simulink model "REFvsFI"  (R2023a)
settings: Solver=FixedStepAuto  StartTime=0.0  StopTime=T  RelTol=1e-3  EnableMultiTasking=on
values from neighbouring files (symbols this model uses):
  Ts = 1    [TestDataGen.m]
libraries: My_FI_Operations x114, simulink x2
(part 1 of 5)
settings Model: FPTShortcutValueString='{{},{''BaselineRun'',1,1,1,''BaselineRun'','''',{},''M'',''D'',''''}}'  Creator=kavru  LastModifiedBy=kolbe
settings OptimizationCC: BlockReduction=off  ConditionallyExecuteInputs=off
settings DebuggingCC: SignalRangeChecking=warning  SingleTaskRateTransMsg=error  UnconnectedInputMsg=warning  UnconnectedOutputMsg=warning  UnconnectedLineMsg=warning
settings ModelReferenceCC: EnableRefExpFcnMdlSchedulingChecks=on
settings RTWCC: DLArmComputeVersion=19.05

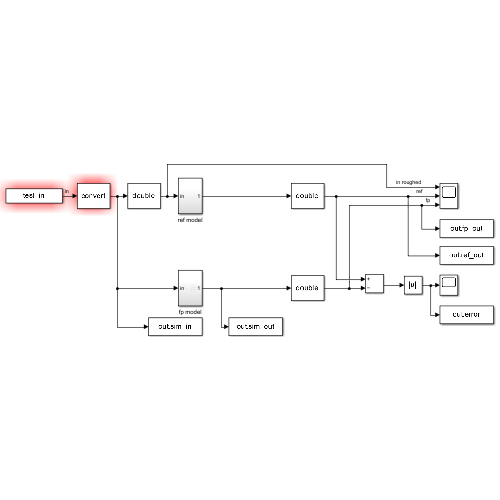
[thumbnail: Simulink's stored preview of the top-level diagram]
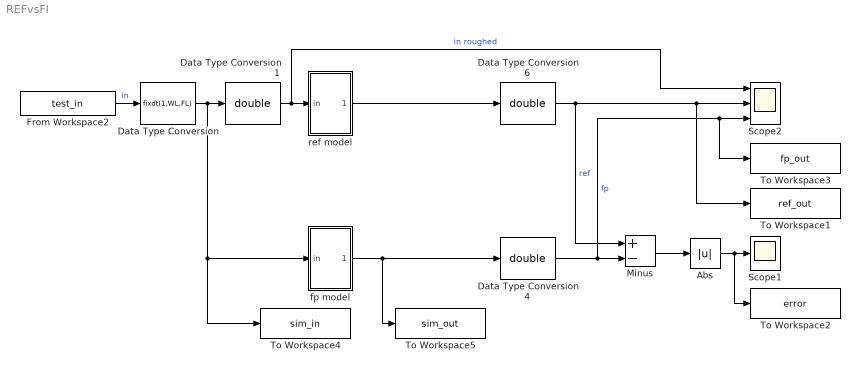
== system REFvsFI ==
  Abs : Abs  SaturateOnIntegerOverflow=off
  Data Type Conversion : DataTypeConversion  OutDataTypeStr=fixdt(1,WL,FL)  RndMeth=Nearest
  Data Type Conversion1 : DataTypeConversion  OutDataTypeStr=double  RndMeth=Nearest  SaturateOnIntegerOverflow=off
  Data Type Conversion4 : DataTypeConversion  OutDataTypeStr=double  RndMeth=Nearest  SaturateOnIntegerOverflow=off
  Data Type Conversion6 : DataTypeConversion  OutDataTypeStr=double  RndMeth=Nearest  SaturateOnIntegerOverflow=off
  From Workspace2 : FromWorkspace  VariableName=test_in  OutDataTypeStr=double  SampleTime=Ts
  Minus : Sum  Inputs=+-
  Scope1 : Scope
  Scope2 : Scope  NumInputPorts=3
  To Workspace1 : ToWorkspace  VariableName=ref_out  SaveFormat=Timeseries  SampleTime=-1
  To Workspace2 : ToWorkspace  VariableName=error  SaveFormat=Timeseries  SampleTime=-1
  To Workspace3 : ToWorkspace  VariableName=fp_out  SaveFormat=Timeseries  SampleTime=-1
  To Workspace4 : ToWorkspace  VariableName=sim_in  SaveFormat=Timeseries  SampleTime=-1
  To Workspace5 : ToWorkspace  VariableName=sim_out  SaveFormat=Timeseries  SampleTime=-1
  fp model : Subsystem
  ref model : Subsystem
  wires:
  From Workspace2/1 -> Data Type Conversion/1  "in"
  Minus/1 -> Abs/1
  Abs/1 -> Scope1/1, To Workspace2/1
  fp model/1(Out1) -> To Workspace5/1, Data Type Conversion4/1
  Data Type Conversion4/1 -> Minus/2, To Workspace3/1, Scope2/3  "fp"
  Data Type Conversion6/1 -> Scope2/2, To Workspace1/1, Minus/1  "ref"
  Data Type Conversion1/1 -> Scope2/1, ref model/1(in)  "in roughed"
  Data Type Conversion/1 -> To Workspace4/1, fp model/1(in), Data Type Conversion1/1
  ref model/1(Out1) -> Data Type Conversion6/1

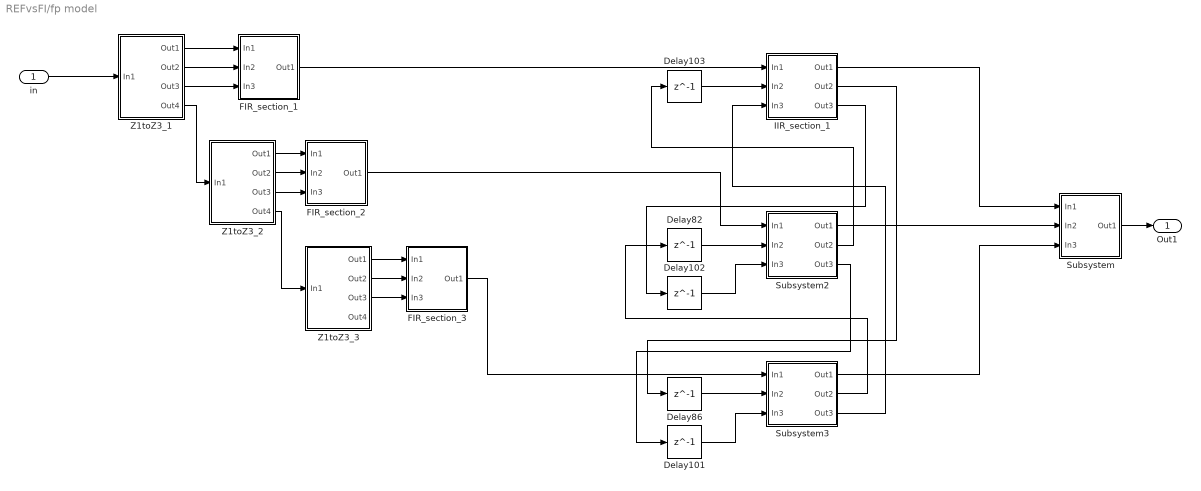
== system REFvsFI/fp model ==
  in : Inport
  Delay{82,86,101..103} (5 alike) : Delay  DelayLength=1  SampleTime=3*Ts
  FIR_section_1 : Subsystem
  FIR_section_2 : Subsystem
  FIR_section_3 : Subsystem
  IIR_section_1 : Subsystem
  Subsystem : Subsystem
  Subsystem2 : Subsystem
  Subsystem3 : Subsystem
  Z1toZ3_1 : Subsystem
  Z1toZ3_2 : Subsystem
  Z1toZ3_3 : Subsystem
  Out1 : Outport
  wires:
  in/1 -> Z1toZ3_1/1(In1)
  Z1toZ3_1/4(Out4) -> Z1toZ3_2/1(In1)
  Z1toZ3_2/4(Out4) -> Z1toZ3_3/1(In1)
  Z1toZ3_1/1(Out1) -> FIR_section_1/1(In1)
  Z1toZ3_1/2(Out2) -> FIR_section_1/2(In2)
  Z1toZ3_1/3(Out3) -> FIR_section_1/3(In3)
  Z1toZ3_2/1(Out1) -> FIR_section_2/1(In1)
  Z1toZ3_2/2(Out2) -> FIR_section_2/2(In2)
  Z1toZ3_2/3(Out3) -> FIR_section_2/3(In3)
  Z1toZ3_3/1(Out1) -> FIR_section_3/1(In1)
  Z1toZ3_3/2(Out2) -> FIR_section_3/2(In2)
  Z1toZ3_3/3(Out3) -> FIR_section_3/3(In3)
  Subsystem/1(Out1) -> Out1/1
  FIR_section_1/1(Out1) -> IIR_section_1/1(In1)
  Delay103/1 -> IIR_section_1/2(In2)
  IIR_section_1/2(Out2) -> Delay86/1
  IIR_section_1/1(Out1) -> Subsystem/1(In1)
  IIR_section_1/3(Out3) -> Delay102/1
  FIR_section_2/1(Out1) -> Subsystem2/1(In1)
  Delay102/1 -> Subsystem2/3(In3)
  Delay82/1 -> Subsystem2/2(In2)
  Subsystem2/1(Out1) -> Subsystem/2(In2)
  Subsystem2/2(Out2) -> Delay103/1
  Subsystem2/3(Out3) -> Delay101/1
  Delay86/1 -> Subsystem3/2(In2)
  Delay101/1 -> Subsystem3/3(In3)
  FIR_section_3/1(Out1) -> Subsystem3/1(In1)
  Subsystem3/3(Out3) -> IIR_section_1/3(In3)
  Subsystem3/1(Out1) -> Subsystem/3(In3)
  Subsystem3/2(Out2) -> Delay82/1
